simulink model "Mophong1"  (R2023a)
settings: Solver=VariableStepAuto  StartTime=0.0  StopTime=10.0  RelTol=1e-3
values from neighbouring files (symbols this model uses):
  Kp1 = cp1*wL    [Code.m]
  position = 7    [Code.m]
  velocity = 7    [Code.m]
libraries: simulink x1
settings Model: Creator=admin  LastModifiedBy=admin

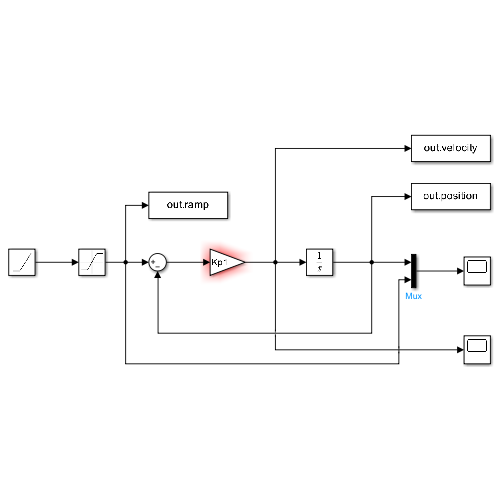
[thumbnail: Simulink's stored preview of the top-level diagram]
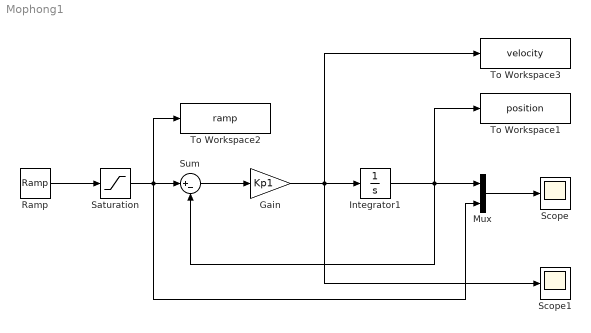
== system Mophong1 ==
  Gain : Gain  Gain=Kp1
  Integrator1 : Integrator
  Mux : Mux  Inputs=2
  Ramp : simulink/Sources/Ramp  slope=velocity  start=0  InitialOutput=0
  Saturation : Saturate  UpperLimit=position  LowerLimit=0
  Scope : Scope
  Scope1 : Scope
  Sum : Sum  Inputs=|+-
  To Workspace1 : ToWorkspace  VariableName=position  SaveFormat=Timeseries  SampleTime=-1
  To Workspace2 : ToWorkspace  VariableName=ramp  SaveFormat=Timeseries  SampleTime=-1
  To Workspace3 : ToWorkspace  VariableName=velocity  SaveFormat=Timeseries  SampleTime=-1
  wires:
  Integrator1/1 -> Mux/1, To Workspace1/1, Sum/2
  Saturation/1 -> Mux/2, To Workspace2/1, Sum/1
  Ramp/1 -> Saturation/1
  Sum/1 -> Gain/1
  Mux/1 -> Scope/1
  Gain/1 -> Scope1/1, To Workspace3/1, Integrator1/1
